simulink library "mwbs_robotSensors_lib"  (R2020b)
settings: Solver=VariableStepAuto  StartTime=0.0  StopTime=10.0  RelTol=1e-3
libraries: WBToolboxLibrary x3
settings Model: Creator=nunoguedelha  LastModifiedBy=nunoguedelha

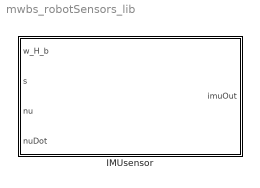
== system mwbs_robotSensors_lib ==
  IMUsensor : Subsystem  mask(IMUsensor){frameName='frame'}
      mask prompts: frameName "Frame name"
      mask help:
      | This block computes the typical outputs of an IMU from the floating base and joints kinematics.
      |
      | Assuming DoFs is the number of internal degrees of freedom of the robot:
      |
      | Input:
      |   - w_H_b: Base pose, 4x4 matrix representing the homogenous transformation between the the base frame and the world frame.
      |   - s: Joint configuration, vector of size DoFs, representing the configuration of the joints.
      |   - nu: Base and joints velocities: Vector of size 6 representing the linear and angular velocity of the base frame, concatenated with a vector of size DoFs, representing the velocity of the joints.
      |   - nuDot: Base and joints accelerations: Vector of size 6 representing the linear and angular acceleration of the base frame, concatenated with a vector of size DoFs, representing the acceleration of the joints.
      |
      | Output:
      |   The sensor frame orientation, linear acceleration and angular velocity w.r.t. the inertial (world) frame. Linear acceleration and angular velocity are expressed in the world frame.
      |   - w_rollPitchYaw: roll, pitch, yaw Euler angles in rad.
      |   - w_linAcc: Proper linear acceleration in m/s^2.
      |   - w_omega: Angular velocity in rad/s.
      |   - imuOut: A [12x1] 1-D vector concatenating the previous three outputs and a placeholder for other measurements (e.g. magnetometer).
      |      [roll,pitch,yaw,accx,accy,accz,omegax,omegay,omegaz,0,0,0]'.
      |
      | Parameters:
      |   - Frame name: the name of the IMU frame. It should be specified in the URDF model.
      mask init:
      | % WBBlock Initialization
      | % ======================
      | 
      | try
      |     [configBlockAbsName, WBTConfig] = WBToolbox.BlockInitialization(gcb, gcs);
      |     robot_NDOF = numel(WBTConfig.ControlledJoints);
      |     GRAVITY_VECTOR = WBTConfig.GravityVector(:);
      |     clear WBTConfig;
      | catch
      | end
      mask DialogControl toggleHighlighting Prompt: Toggle Config Block Highlighting
      mask DialogControl toggleHighlighting Callback:
      | [configBlock, ~] = WBToolbox.BlockInitialization(gcb, gcs);
      | 
      | try
      |     if (strcmp(get_param(configBlock,'HiliteAncestors'),'none'))
      |         hilite_system(configBlock,'find');
      |     else
      |         hilite_system(configBlock,'none');
      |     end
      | catch
      |     error('[%s:ShowConfigBlock:Callback] Failed to process config block name: %s',gcb,configBlock);
      | end
      | 
      | clear configBlock
      mask Display: disp('IMU')

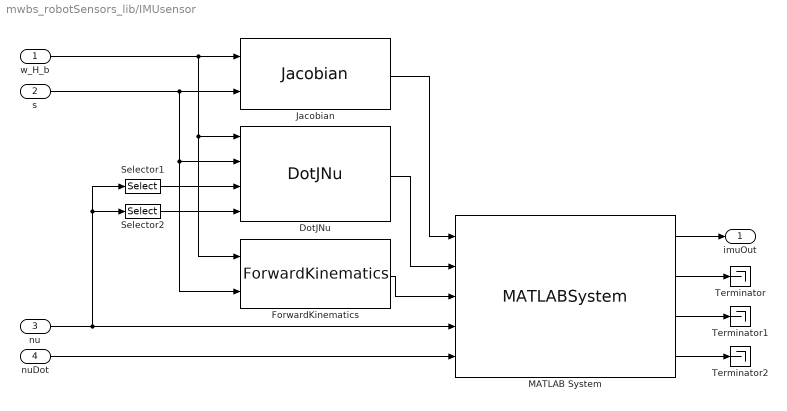
== system mwbs_robotSensors_lib/IMUsensor ==
  w_H_b : Inport
  s : Inport  Port=2
  nu : Inport  Port=3
  nuDot : Inport  Port=4
  DotJNu : WBToolboxLibrary/Model/Jacobians/DotJNu  frameName=frameName
      settings: SourceProductName=WholeBodyToolbox
  ForwardKinematics : WBToolboxLibrary/Model/Kinematics/ForwardKinematics  frameName=frameName
      settings: SourceProductName=WholeBodyToolbox
  Jacobian : WBToolboxLibrary/Model/Jacobians/Jacobian  frameName=frameName
      settings: SourceProductName=WholeBodyToolbox
  MATLAB System : MATLABSystem  System=mwbs.RobotSensors.IMUsensor.IMUsensorProc  GRAVITY_VECTOR=GRAVITY_VECTOR  SimulateUsing=Code generation
      mask Type: mwbs.RobotSensors.IMUsensor.IMUsensorProc
      mask Display:
      | disp('IMUsensorProc');
      | port_label('input',1,'Jimu');
      | port_label('input',2,'JimuDotNu');
      | port_label('input',3,'w_H_imu');
      | port_label('input',4,'nu');
      | port_label('input',5,'nudot');
      | port_label('output',1,'imuOut');
      | port_label('output',2,'w_omega');
      | port_label('output',3,'w_linAcc');
      | port_label('output',4,'w_rollPitchYaw');
  Selector1 : Selector  IndexOptions=Index vector (dialog)  Indices=[1:6]  OutputSizes=1
  Selector2 : Selector  IndexOptions=Starting index (dialog)  Indices=7  OutputSizes=robot_NDOF
  Terminator : Terminator
  Terminator1 : Terminator
  Terminator2 : Terminator
  imuOut : Outport
  wires:
  MATLAB System/3 -> Terminator1/1
  MATLAB System/1 -> imuOut/1
  MATLAB System/2 -> Terminator/1
  s/1 -> DotJNu/2, ForwardKinematics/2, Jacobian/2
  nu/1 -> Selector2/1, Selector1/1, MATLAB System/4
  nuDot/1 -> MATLAB System/5
  Jacobian/1 -> MATLAB System/1
  MATLAB System/4 -> Terminator2/1
  ForwardKinematics/1 -> MATLAB System/3
  w_H_b/1 -> DotJNu/1, ForwardKinematics/1, Jacobian/1
  DotJNu/1 -> MATLAB System/2
  Selector1/1 -> DotJNu/3
  Selector2/1 -> DotJNu/4
